simulink model "Pendulum_param_sim"  (Simulink 8.9)
settings: Solver=ode3  StartTime=0.0  StopTime=100  FixedStep=T  RelTol=1e-3  EnableMultiTasking=on
undefined symbols (not defined in the file): angle_0, c1_hat, c2_hat, g, l_hat, m
settings Model: Creator=Stefan  LastModifiedBy=Administrator
settings OptimizationCC: ExpressionDepthLimit=2147483647
settings DebuggingCC: SolverPrmCheckMsg=warning  AllowSymbolicDim=off

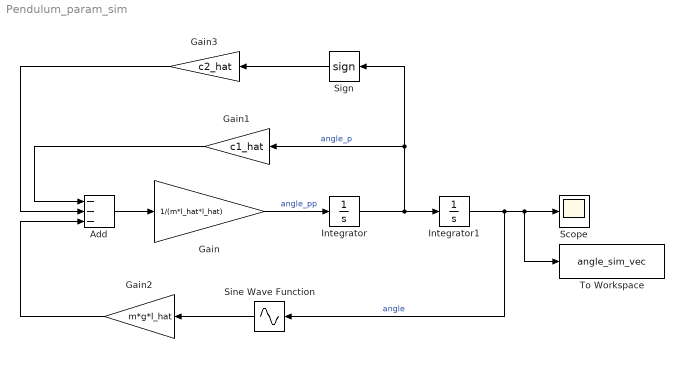
== system Pendulum_param_sim ==
  Add : Sum  Inputs=---
  Gain : Gain  Gain=1/(m*l_hat*l_hat)
  Gain1 : Gain  Gain=c1_hat
  Gain2 : Gain  Gain=m*g*l_hat
  Gain3 : Gain  Gain=c2_hat
  Integrator : Integrator
  Integrator1 : Integrator  InitialCondition=angle_0
  Scope : Scope
  Sign : Signum
  Sine Wave Function : Sin  TimeSource=Use external signal  SampleTime=0
  To Workspace : ToWorkspace  VariableName=angle_sim_vec  SaveFormat=Structure  SampleTime=-1
  wires:
  Gain/1 -> Integrator/1  "angle_pp"
  Add/1 -> Gain/1
  Integrator/1 -> Integrator1/1, Sign/1, Gain1/1  "angle_p"
  Gain1/1 -> Add/1
  Sine Wave Function/1 -> Gain2/1
  Integrator1/1 -> Sine Wave Function/1, Scope/1, To Workspace/1  "angle"
  Gain3/1 -> Add/2
  Gain2/1 -> Add/3
  Sign/1 -> Gain3/1
